simulink model "Distribution"  (R2018b)
settings: Solver=ode45  StartTime=0.0  StopTime=100  RelTol=1e-3
libraries: simeventslib x20
(part 2 of 2)

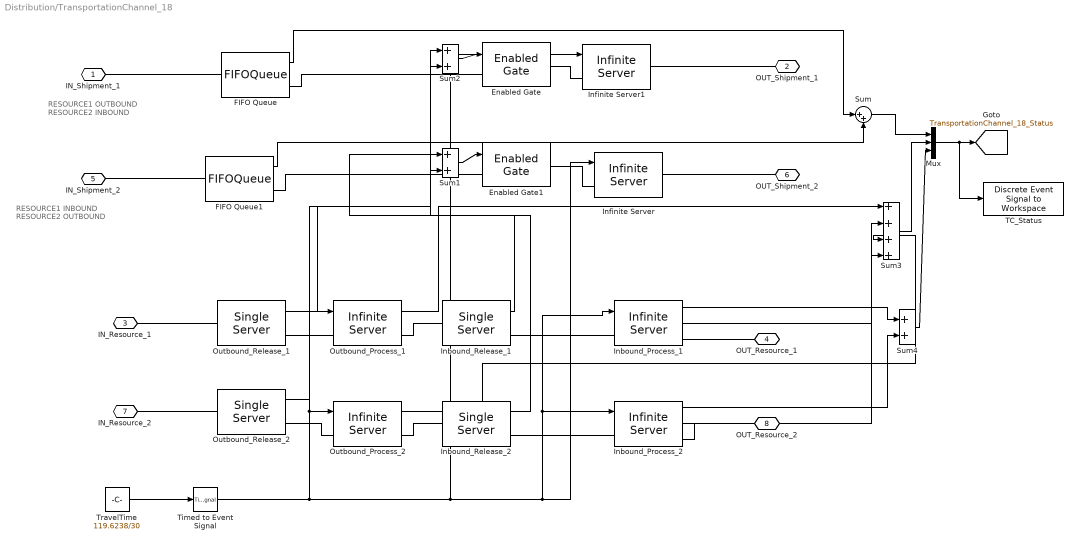
== system Distribution/TransportationChannel_18 ==
  note: RESOURCE1 OUTBOUND
      | RESOURCE2 INBOUND
  note: RESOURCE1 INBOUND
      | RESOURCE2 OUTBOUND
  Enabled Gate : EnabledGate
  Enabled Gate1 : EnabledGate
  FIFO Queue : FIFOQueue  Capacity=inf  StatNumberInBlock=on
      settings: OutputPortMap=o1
  FIFO Queue1 : FIFOQueue  Capacity=inf  StatNumberInBlock=on
      settings: OutputPortMap=o1
  Inbound_Process_1 : InfiniteServer  ServiceTimeFrom=Signal port t  ServiceTime=(76.7)/30  StatNumberDeparted=on  StatNumberInBlock=on
      settings: OutputPortMap=o0,o1
  Inbound_Process_2 : InfiniteServer  ServiceTimeFrom=Signal port t  ServiceTime=(76.7)/30  StatNumberDeparted=on  StatNumberInBlock=on
      settings: OutputPortMap=o0,o1
  Inbound_Release_1 : SingleServer  ServiceTime=0  StatNumberInBlock=on
      settings: OutputPortMap=o1
  Inbound_Release_2 : SingleServer  ServiceTime=0  StatNumberInBlock=on
      settings: OutputPortMap=o1
  Infinite Server : InfiniteServer  ServiceTimeFrom=Signal port t  ServiceTime=(76.7)/30
  Infinite Server1 : InfiniteServer  ServiceTimeFrom=Signal port t  ServiceTime=(76.7)/30
  Mux : Mux  Inputs=3
  Outbound_Process_1 : InfiniteServer  ServiceTimeFrom=Signal port t  ServiceTime=(76.7)/30  StatNumberInBlock=on
      settings: OutputPortMap=o1
  Outbound_Process_2 : InfiniteServer  ServiceTimeFrom=Signal port t  ServiceTime=(76.7)/30  StatNumberInBlock=on
      settings: OutputPortMap=o1
  Outbound_Release_1 : SingleServer  ServiceTime=0  StatNumberInBlock=on
      settings: OutputPortMap=o1
  Outbound_Release_2 : SingleServer  ServiceTime=0  StatNumberInBlock=on
      settings: OutputPortMap=o1
  Sum{,1..2,4} (4 alike) : Sum  Inputs=|++
  Sum3 : Sum  Inputs=|++++
  TC_Status : simeventslib/SimEvents Sinks/Discrete Event Signal to Workspace  VariableName=TransportationChannel_18_Status  SaveFormat=Structure With Time  isMonitorOnly=off  isRecordIC=off
      settings: SourceProductName=SimEvents  SourceProductBaseCode=SE
  Timed to Event Signal : TimedToEventSignal
  TravelTime : Constant  Value=119.6238/30
  IN_Shipment_1 : PMIOPort  Side=Left
  OUT_Shipment_1 : PMIOPort  Port=2  Side=Right
  IN_Resource_1 : PMIOPort  Port=3  Side=Left
  OUT_Resource_1 : PMIOPort  Port=4  Side=Right
  IN_Shipment_2 : PMIOPort  Port=5  Side=Left
  OUT_Shipment_2 : PMIOPort  Port=6  Side=Right
  IN_Resource_2 : PMIOPort  Port=7  Side=Left
  OUT_Resource_2 : PMIOPort  Port=8  Side=Right
  tag scope: TransportationChannel_18_Status=global
  wires:
  Sum4/1 -> Mux/3
  Inbound_Process_2/1 -> Sum4/2
  Inbound_Process_1/1 -> Sum4/1
  Inbound_Process_2/2 -> Sum3/4
  Outbound_Process_2/1 -> Sum3/3
  Inbound_Process_1/2 -> Sum3/2
  Outbound_Process_1/1 -> Sum3/1
  Sum3/1 -> Mux/2
  Sum/1 -> Mux/1
  Mux/1 -> TC_Status/1, [TransportationChannel_18_Status]
  Inbound_Release_2/1 -> Sum2/2
  Outbound_Release_1/1 -> Sum2/1
  Sum2/1 -> Enabled Gate/1
  Inbound_Release_1/1 -> Sum1/1
  Outbound_Release_2/1 -> Sum1/2
  Sum1/1 -> Enabled Gate1/1
  Timed to Event Signal/1 -> Outbound_Process_2/1, Outbound_Process_1/1, Infinite Server1/1, Inbound_Process_2/1, Inbound_Process_1/1, Infinite Server/1
  TravelTime/1 -> Timed to Event Signal/1
  FIFO Queue/1 -> Sum/1
  FIFO Queue1/1 -> Sum/2
  connections:
  Inbound_Process_1/RConn1 -- OUT_Resource_1/RConn1
  Outbound_Process_1/RConn1 -- Inbound_Release_1/LConn1
  Inbound_Release_1/RConn1 -- Inbound_Process_1/LConn1
  Outbound_Release_1/RConn1 -- Outbound_Process_1/LConn1
  Inbound_Process_2/RConn1 -- OUT_Resource_2/RConn1
  Inbound_Release_2/RConn1 -- Inbound_Process_2/LConn1
  Outbound_Process_2/RConn1 -- Inbound_Release_2/LConn1
  Outbound_Release_2/RConn1 -- Outbound_Process_2/LConn1
  IN_Resource_2/RConn1 -- Outbound_Release_2/LConn1
  Infinite Server1/RConn1 -- OUT_Shipment_1/RConn1
  Enabled Gate/RConn1 -- Infinite Server1/LConn1
  Infinite Server/LConn1 -- Enabled Gate1/RConn1
  OUT_Shipment_2/RConn1 -- Infinite Server/RConn1
  IN_Resource_1/RConn1 -- Outbound_Release_1/LConn1
  IN_Shipment_2/RConn1 -- FIFO Queue1/LConn1
  IN_Shipment_1/RConn1 -- FIFO Queue/LConn1
  Enabled Gate1/LConn1 -- FIFO Queue1/RConn1
  FIFO Queue/RConn1 -- Enabled Gate/LConn1

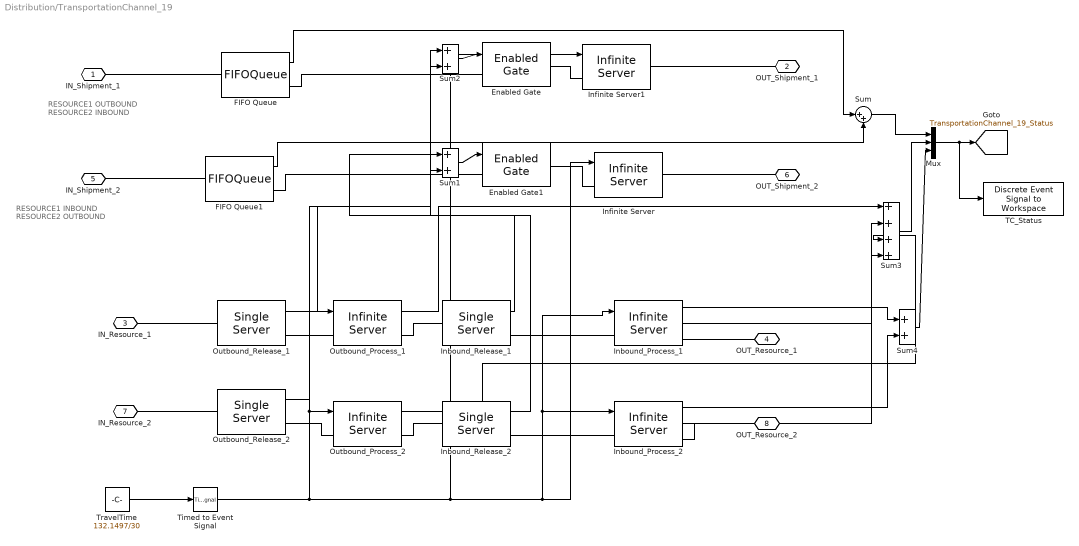
== system Distribution/TransportationChannel_19 ==
  note: RESOURCE1 OUTBOUND
      | RESOURCE2 INBOUND
  note: RESOURCE1 INBOUND
      | RESOURCE2 OUTBOUND
  Enabled Gate : EnabledGate
  Enabled Gate1 : EnabledGate
  FIFO Queue : FIFOQueue  Capacity=inf  StatNumberInBlock=on
      settings: OutputPortMap=o1
  FIFO Queue1 : FIFOQueue  Capacity=inf  StatNumberInBlock=on
      settings: OutputPortMap=o1
  Inbound_Process_1 : InfiniteServer  ServiceTimeFrom=Signal port t  ServiceTime=(76.7)/30  StatNumberDeparted=on  StatNumberInBlock=on
      settings: OutputPortMap=o0,o1
  Inbound_Process_2 : InfiniteServer  ServiceTimeFrom=Signal port t  ServiceTime=(76.7)/30  StatNumberDeparted=on  StatNumberInBlock=on
      settings: OutputPortMap=o0,o1
  Inbound_Release_1 : SingleServer  ServiceTime=0  StatNumberInBlock=on
      settings: OutputPortMap=o1
  Inbound_Release_2 : SingleServer  ServiceTime=0  StatNumberInBlock=on
      settings: OutputPortMap=o1
  Infinite Server : InfiniteServer  ServiceTimeFrom=Signal port t  ServiceTime=(76.7)/30
  Infinite Server1 : InfiniteServer  ServiceTimeFrom=Signal port t  ServiceTime=(76.7)/30
  Mux : Mux  Inputs=3
  Outbound_Process_1 : InfiniteServer  ServiceTimeFrom=Signal port t  ServiceTime=(76.7)/30  StatNumberInBlock=on
      settings: OutputPortMap=o1
  Outbound_Process_2 : InfiniteServer  ServiceTimeFrom=Signal port t  ServiceTime=(76.7)/30  StatNumberInBlock=on
      settings: OutputPortMap=o1
  Outbound_Release_1 : SingleServer  ServiceTime=0  StatNumberInBlock=on
      settings: OutputPortMap=o1
  Outbound_Release_2 : SingleServer  ServiceTime=0  StatNumberInBlock=on
      settings: OutputPortMap=o1
  Sum{,1..2,4} (4 alike) : Sum  Inputs=|++
  Sum3 : Sum  Inputs=|++++
  TC_Status : simeventslib/SimEvents Sinks/Discrete Event Signal to Workspace  VariableName=TransportationChannel_19_Status  SaveFormat=Structure With Time  isMonitorOnly=off  isRecordIC=off
      settings: SourceProductName=SimEvents  SourceProductBaseCode=SE
  Timed to Event Signal : TimedToEventSignal
  TravelTime : Constant  Value=132.1497/30
  IN_Shipment_1 : PMIOPort  Side=Left
  OUT_Shipment_1 : PMIOPort  Port=2  Side=Right
  IN_Resource_1 : PMIOPort  Port=3  Side=Left
  OUT_Resource_1 : PMIOPort  Port=4  Side=Right
  IN_Shipment_2 : PMIOPort  Port=5  Side=Left
  OUT_Shipment_2 : PMIOPort  Port=6  Side=Right
  IN_Resource_2 : PMIOPort  Port=7  Side=Left
  OUT_Resource_2 : PMIOPort  Port=8  Side=Right
  tag scope: TransportationChannel_19_Status=global
  wires:
  Sum4/1 -> Mux/3
  Inbound_Process_2/1 -> Sum4/2
  Inbound_Process_1/1 -> Sum4/1
  Inbound_Process_2/2 -> Sum3/4
  Outbound_Process_2/1 -> Sum3/3
  Inbound_Process_1/2 -> Sum3/2
  Outbound_Process_1/1 -> Sum3/1
  Sum3/1 -> Mux/2
  Sum/1 -> Mux/1
  Mux/1 -> TC_Status/1, [TransportationChannel_19_Status]
  Inbound_Release_2/1 -> Sum2/2
  Outbound_Release_1/1 -> Sum2/1
  Sum2/1 -> Enabled Gate/1
  Inbound_Release_1/1 -> Sum1/1
  Outbound_Release_2/1 -> Sum1/2
  Sum1/1 -> Enabled Gate1/1
  Timed to Event Signal/1 -> Outbound_Process_2/1, Outbound_Process_1/1, Infinite Server1/1, Inbound_Process_2/1, Inbound_Process_1/1, Infinite Server/1
  TravelTime/1 -> Timed to Event Signal/1
  FIFO Queue/1 -> Sum/1
  FIFO Queue1/1 -> Sum/2
  connections:
  Inbound_Process_1/RConn1 -- OUT_Resource_1/RConn1
  Outbound_Process_1/RConn1 -- Inbound_Release_1/LConn1
  Inbound_Release_1/RConn1 -- Inbound_Process_1/LConn1
  Outbound_Release_1/RConn1 -- Outbound_Process_1/LConn1
  Inbound_Process_2/RConn1 -- OUT_Resource_2/RConn1
  Inbound_Release_2/RConn1 -- Inbound_Process_2/LConn1
  Outbound_Process_2/RConn1 -- Inbound_Release_2/LConn1
  Outbound_Release_2/RConn1 -- Outbound_Process_2/LConn1
  IN_Resource_2/RConn1 -- Outbound_Release_2/LConn1
  Infinite Server1/RConn1 -- OUT_Shipment_1/RConn1
  Enabled Gate/RConn1 -- Infinite Server1/LConn1
  Infinite Server/LConn1 -- Enabled Gate1/RConn1
  OUT_Shipment_2/RConn1 -- Infinite Server/RConn1
  IN_Resource_1/RConn1 -- Outbound_Release_1/LConn1
  IN_Shipment_2/RConn1 -- FIFO Queue1/LConn1
  IN_Shipment_1/RConn1 -- FIFO Queue/LConn1
  Enabled Gate1/LConn1 -- FIFO Queue1/RConn1
  FIFO Queue/RConn1 -- Enabled Gate/LConn1

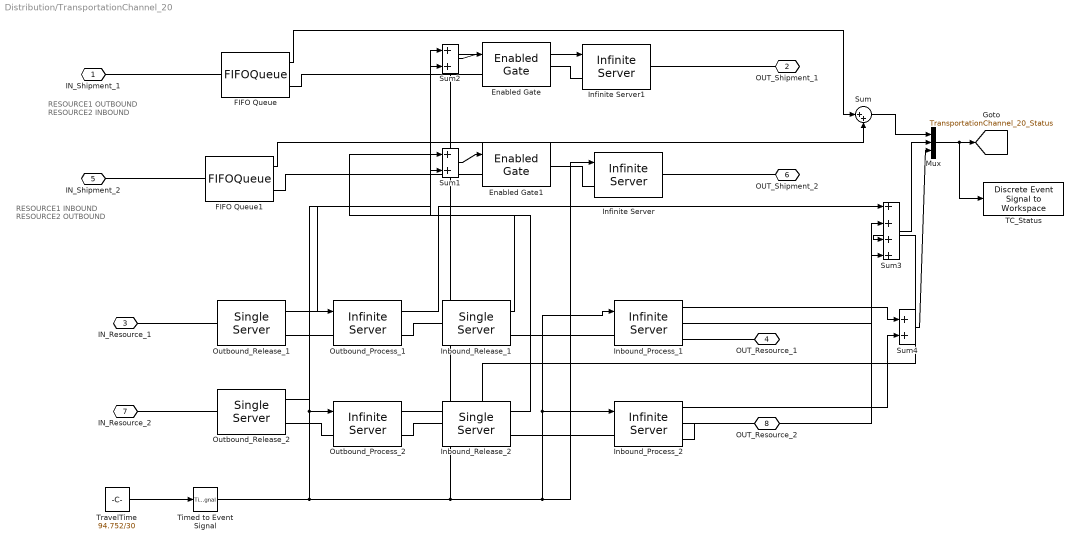
== system Distribution/TransportationChannel_20 ==
  note: RESOURCE1 OUTBOUND
      | RESOURCE2 INBOUND
  note: RESOURCE1 INBOUND
      | RESOURCE2 OUTBOUND
  Enabled Gate : EnabledGate
  Enabled Gate1 : EnabledGate
  FIFO Queue : FIFOQueue  Capacity=inf  StatNumberInBlock=on
      settings: OutputPortMap=o1
  FIFO Queue1 : FIFOQueue  Capacity=inf  StatNumberInBlock=on
      settings: OutputPortMap=o1
  Inbound_Process_1 : InfiniteServer  ServiceTimeFrom=Signal port t  ServiceTime=(76.7)/30  StatNumberDeparted=on  StatNumberInBlock=on
      settings: OutputPortMap=o0,o1
  Inbound_Process_2 : InfiniteServer  ServiceTimeFrom=Signal port t  ServiceTime=(76.7)/30  StatNumberDeparted=on  StatNumberInBlock=on
      settings: OutputPortMap=o0,o1
  Inbound_Release_1 : SingleServer  ServiceTime=0  StatNumberInBlock=on
      settings: OutputPortMap=o1
  Inbound_Release_2 : SingleServer  ServiceTime=0  StatNumberInBlock=on
      settings: OutputPortMap=o1
  Infinite Server : InfiniteServer  ServiceTimeFrom=Signal port t  ServiceTime=(76.7)/30
  Infinite Server1 : InfiniteServer  ServiceTimeFrom=Signal port t  ServiceTime=(76.7)/30
  Mux : Mux  Inputs=3
  Outbound_Process_1 : InfiniteServer  ServiceTimeFrom=Signal port t  ServiceTime=(76.7)/30  StatNumberInBlock=on
      settings: OutputPortMap=o1
  Outbound_Process_2 : InfiniteServer  ServiceTimeFrom=Signal port t  ServiceTime=(76.7)/30  StatNumberInBlock=on
      settings: OutputPortMap=o1
  Outbound_Release_1 : SingleServer  ServiceTime=0  StatNumberInBlock=on
      settings: OutputPortMap=o1
  Outbound_Release_2 : SingleServer  ServiceTime=0  StatNumberInBlock=on
      settings: OutputPortMap=o1
  Sum{,1..2,4} (4 alike) : Sum  Inputs=|++
  Sum3 : Sum  Inputs=|++++
  TC_Status : simeventslib/SimEvents Sinks/Discrete Event Signal to Workspace  VariableName=TransportationChannel_20_Status  SaveFormat=Structure With Time  isMonitorOnly=off  isRecordIC=off
      settings: SourceProductName=SimEvents  SourceProductBaseCode=SE
  Timed to Event Signal : TimedToEventSignal
  TravelTime : Constant  Value=94.752/30
  IN_Shipment_1 : PMIOPort  Side=Left
  OUT_Shipment_1 : PMIOPort  Port=2  Side=Right
  IN_Resource_1 : PMIOPort  Port=3  Side=Left
  OUT_Resource_1 : PMIOPort  Port=4  Side=Right
  IN_Shipment_2 : PMIOPort  Port=5  Side=Left
  OUT_Shipment_2 : PMIOPort  Port=6  Side=Right
  IN_Resource_2 : PMIOPort  Port=7  Side=Left
  OUT_Resource_2 : PMIOPort  Port=8  Side=Right
  tag scope: TransportationChannel_20_Status=global
  wires:
  Sum4/1 -> Mux/3
  Inbound_Process_2/1 -> Sum4/2
  Inbound_Process_1/1 -> Sum4/1
  Inbound_Process_2/2 -> Sum3/4
  Outbound_Process_2/1 -> Sum3/3
  Inbound_Process_1/2 -> Sum3/2
  Outbound_Process_1/1 -> Sum3/1
  Sum3/1 -> Mux/2
  Sum/1 -> Mux/1
  Mux/1 -> TC_Status/1, [TransportationChannel_20_Status]
  Inbound_Release_2/1 -> Sum2/2
  Outbound_Release_1/1 -> Sum2/1
  Sum2/1 -> Enabled Gate/1
  Inbound_Release_1/1 -> Sum1/1
  Outbound_Release_2/1 -> Sum1/2
  Sum1/1 -> Enabled Gate1/1
  Timed to Event Signal/1 -> Outbound_Process_2/1, Outbound_Process_1/1, Infinite Server1/1, Inbound_Process_2/1, Inbound_Process_1/1, Infinite Server/1
  TravelTime/1 -> Timed to Event Signal/1
  FIFO Queue/1 -> Sum/1
  FIFO Queue1/1 -> Sum/2
  connections:
  Inbound_Process_1/RConn1 -- OUT_Resource_1/RConn1
  Outbound_Process_1/RConn1 -- Inbound_Release_1/LConn1
  Inbound_Release_1/RConn1 -- Inbound_Process_1/LConn1
  Outbound_Release_1/RConn1 -- Outbound_Process_1/LConn1
  Inbound_Process_2/RConn1 -- OUT_Resource_2/RConn1
  Inbound_Release_2/RConn1 -- Inbound_Process_2/LConn1
  Outbound_Process_2/RConn1 -- Inbound_Release_2/LConn1
  Outbound_Release_2/RConn1 -- Outbound_Process_2/LConn1
  IN_Resource_2/RConn1 -- Outbound_Release_2/LConn1
  Infinite Server1/RConn1 -- OUT_Shipment_1/RConn1
  Enabled Gate/RConn1 -- Infinite Server1/LConn1
  Infinite Server/LConn1 -- Enabled Gate1/RConn1
  OUT_Shipment_2/RConn1 -- Infinite Server/RConn1
  IN_Resource_1/RConn1 -- Outbound_Release_1/LConn1
  IN_Shipment_2/RConn1 -- FIFO Queue1/LConn1
  IN_Shipment_1/RConn1 -- FIFO Queue/LConn1
  Enabled Gate1/LConn1 -- FIFO Queue1/RConn1
  FIFO Queue/RConn1 -- Enabled Gate/LConn1

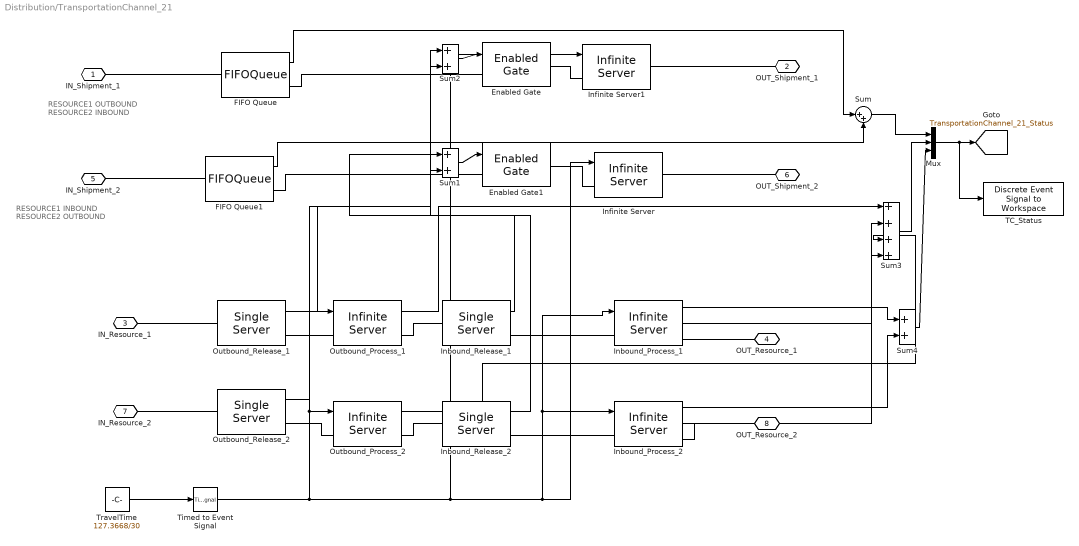
== system Distribution/TransportationChannel_21 ==
  note: RESOURCE1 OUTBOUND
      | RESOURCE2 INBOUND
  note: RESOURCE1 INBOUND
      | RESOURCE2 OUTBOUND
  Enabled Gate : EnabledGate
  Enabled Gate1 : EnabledGate
  FIFO Queue : FIFOQueue  Capacity=inf  StatNumberInBlock=on
      settings: OutputPortMap=o1
  FIFO Queue1 : FIFOQueue  Capacity=inf  StatNumberInBlock=on
      settings: OutputPortMap=o1
  Inbound_Process_1 : InfiniteServer  ServiceTimeFrom=Signal port t  ServiceTime=(76.7)/30  StatNumberDeparted=on  StatNumberInBlock=on
      settings: OutputPortMap=o0,o1
  Inbound_Process_2 : InfiniteServer  ServiceTimeFrom=Signal port t  ServiceTime=(76.7)/30  StatNumberDeparted=on  StatNumberInBlock=on
      settings: OutputPortMap=o0,o1
  Inbound_Release_1 : SingleServer  ServiceTime=0  StatNumberInBlock=on
      settings: OutputPortMap=o1
  Inbound_Release_2 : SingleServer  ServiceTime=0  StatNumberInBlock=on
      settings: OutputPortMap=o1
  Infinite Server : InfiniteServer  ServiceTimeFrom=Signal port t  ServiceTime=(76.7)/30
  Infinite Server1 : InfiniteServer  ServiceTimeFrom=Signal port t  ServiceTime=(76.7)/30
  Mux : Mux  Inputs=3
  Outbound_Process_1 : InfiniteServer  ServiceTimeFrom=Signal port t  ServiceTime=(76.7)/30  StatNumberInBlock=on
      settings: OutputPortMap=o1
  Outbound_Process_2 : InfiniteServer  ServiceTimeFrom=Signal port t  ServiceTime=(76.7)/30  StatNumberInBlock=on
      settings: OutputPortMap=o1
  Outbound_Release_1 : SingleServer  ServiceTime=0  StatNumberInBlock=on
      settings: OutputPortMap=o1
  Outbound_Release_2 : SingleServer  ServiceTime=0  StatNumberInBlock=on
      settings: OutputPortMap=o1
  Sum{,1..2,4} (4 alike) : Sum  Inputs=|++
  Sum3 : Sum  Inputs=|++++
  TC_Status : simeventslib/SimEvents Sinks/Discrete Event Signal to Workspace  VariableName=TransportationChannel_21_Status  SaveFormat=Structure With Time  isMonitorOnly=off  isRecordIC=off
      settings: SourceProductName=SimEvents  SourceProductBaseCode=SE
  Timed to Event Signal : TimedToEventSignal
  TravelTime : Constant  Value=127.3668/30
  IN_Shipment_1 : PMIOPort  Side=Left
  OUT_Shipment_1 : PMIOPort  Port=2  Side=Right
  IN_Resource_1 : PMIOPort  Port=3  Side=Left
  OUT_Resource_1 : PMIOPort  Port=4  Side=Right
  IN_Shipment_2 : PMIOPort  Port=5  Side=Left
  OUT_Shipment_2 : PMIOPort  Port=6  Side=Right
  IN_Resource_2 : PMIOPort  Port=7  Side=Left
  OUT_Resource_2 : PMIOPort  Port=8  Side=Right
  tag scope: TransportationChannel_21_Status=global
  wires:
  Sum4/1 -> Mux/3
  Inbound_Process_2/1 -> Sum4/2
  Inbound_Process_1/1 -> Sum4/1
  Inbound_Process_2/2 -> Sum3/4
  Outbound_Process_2/1 -> Sum3/3
  Inbound_Process_1/2 -> Sum3/2
  Outbound_Process_1/1 -> Sum3/1
  Sum3/1 -> Mux/2
  Sum/1 -> Mux/1
  Mux/1 -> TC_Status/1, [TransportationChannel_21_Status]
  Inbound_Release_2/1 -> Sum2/2
  Outbound_Release_1/1 -> Sum2/1
  Sum2/1 -> Enabled Gate/1
  Inbound_Release_1/1 -> Sum1/1
  Outbound_Release_2/1 -> Sum1/2
  Sum1/1 -> Enabled Gate1/1
  Timed to Event Signal/1 -> Outbound_Process_2/1, Outbound_Process_1/1, Infinite Server1/1, Inbound_Process_2/1, Inbound_Process_1/1, Infinite Server/1
  TravelTime/1 -> Timed to Event Signal/1
  FIFO Queue/1 -> Sum/1
  FIFO Queue1/1 -> Sum/2
  connections:
  Inbound_Process_1/RConn1 -- OUT_Resource_1/RConn1
  Outbound_Process_1/RConn1 -- Inbound_Release_1/LConn1
  Inbound_Release_1/RConn1 -- Inbound_Process_1/LConn1
  Outbound_Release_1/RConn1 -- Outbound_Process_1/LConn1
  Inbound_Process_2/RConn1 -- OUT_Resource_2/RConn1
  Inbound_Release_2/RConn1 -- Inbound_Process_2/LConn1
  Outbound_Process_2/RConn1 -- Inbound_Release_2/LConn1
  Outbound_Release_2/RConn1 -- Outbound_Process_2/LConn1
  IN_Resource_2/RConn1 -- Outbound_Release_2/LConn1
  Infinite Server1/RConn1 -- OUT_Shipment_1/RConn1
  Enabled Gate/RConn1 -- Infinite Server1/LConn1
  Infinite Server/LConn1 -- Enabled Gate1/RConn1
  OUT_Shipment_2/RConn1 -- Infinite Server/RConn1
  IN_Resource_1/RConn1 -- Outbound_Release_1/LConn1
  IN_Shipment_2/RConn1 -- FIFO Queue1/LConn1
  IN_Shipment_1/RConn1 -- FIFO Queue/LConn1
  Enabled Gate1/LConn1 -- FIFO Queue1/RConn1
  FIFO Queue/RConn1 -- Enabled Gate/LConn1

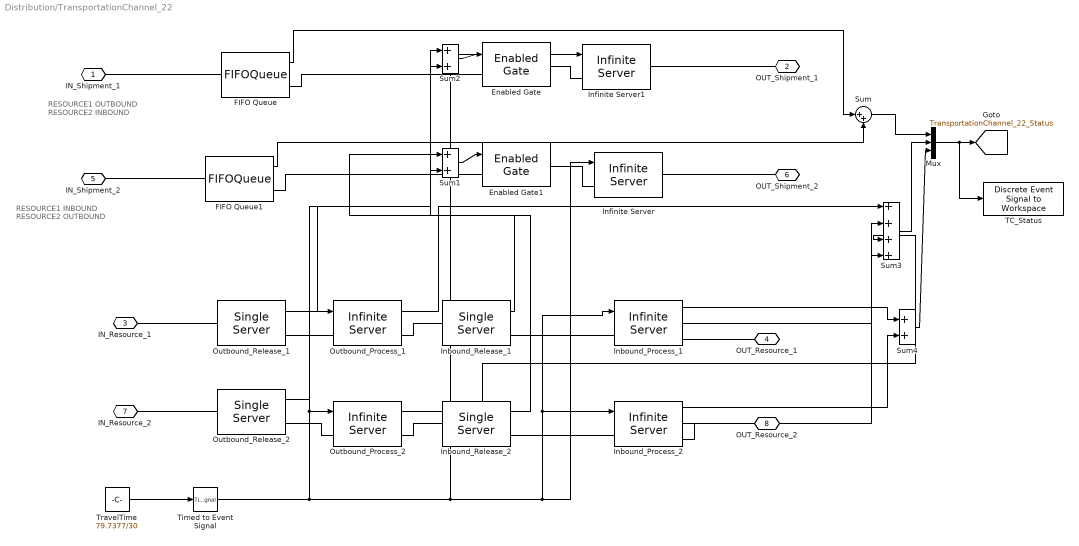
== system Distribution/TransportationChannel_22 ==
  note: RESOURCE1 OUTBOUND
      | RESOURCE2 INBOUND
  note: RESOURCE1 INBOUND
      | RESOURCE2 OUTBOUND
  Enabled Gate : EnabledGate
  Enabled Gate1 : EnabledGate
  FIFO Queue : FIFOQueue  Capacity=inf  StatNumberInBlock=on
      settings: OutputPortMap=o1
  FIFO Queue1 : FIFOQueue  Capacity=inf  StatNumberInBlock=on
      settings: OutputPortMap=o1
  Inbound_Process_1 : InfiniteServer  ServiceTimeFrom=Signal port t  ServiceTime=(76.7)/30  StatNumberDeparted=on  StatNumberInBlock=on
      settings: OutputPortMap=o0,o1
  Inbound_Process_2 : InfiniteServer  ServiceTimeFrom=Signal port t  ServiceTime=(76.7)/30  StatNumberDeparted=on  StatNumberInBlock=on
      settings: OutputPortMap=o0,o1
  Inbound_Release_1 : SingleServer  ServiceTime=0  StatNumberInBlock=on
      settings: OutputPortMap=o1
  Inbound_Release_2 : SingleServer  ServiceTime=0  StatNumberInBlock=on
      settings: OutputPortMap=o1
  Infinite Server : InfiniteServer  ServiceTimeFrom=Signal port t  ServiceTime=(76.7)/30
  Infinite Server1 : InfiniteServer  ServiceTimeFrom=Signal port t  ServiceTime=(76.7)/30
  Mux : Mux  Inputs=3
  Outbound_Process_1 : InfiniteServer  ServiceTimeFrom=Signal port t  ServiceTime=(76.7)/30  StatNumberInBlock=on
      settings: OutputPortMap=o1
  Outbound_Process_2 : InfiniteServer  ServiceTimeFrom=Signal port t  ServiceTime=(76.7)/30  StatNumberInBlock=on
      settings: OutputPortMap=o1
  Outbound_Release_1 : SingleServer  ServiceTime=0  StatNumberInBlock=on
      settings: OutputPortMap=o1
  Outbound_Release_2 : SingleServer  ServiceTime=0  StatNumberInBlock=on
      settings: OutputPortMap=o1
  Sum{,1..2,4} (4 alike) : Sum  Inputs=|++
  Sum3 : Sum  Inputs=|++++
  TC_Status : simeventslib/SimEvents Sinks/Discrete Event Signal to Workspace  VariableName=TransportationChannel_22_Status  SaveFormat=Structure With Time  isMonitorOnly=off  isRecordIC=off
      settings: SourceProductName=SimEvents  SourceProductBaseCode=SE
  Timed to Event Signal : TimedToEventSignal
  TravelTime : Constant  Value=79.7377/30
  IN_Shipment_1 : PMIOPort  Side=Left
  OUT_Shipment_1 : PMIOPort  Port=2  Side=Right
  IN_Resource_1 : PMIOPort  Port=3  Side=Left
  OUT_Resource_1 : PMIOPort  Port=4  Side=Right
  IN_Shipment_2 : PMIOPort  Port=5  Side=Left
  OUT_Shipment_2 : PMIOPort  Port=6  Side=Right
  IN_Resource_2 : PMIOPort  Port=7  Side=Left
  OUT_Resource_2 : PMIOPort  Port=8  Side=Right
  tag scope: TransportationChannel_22_Status=global
  wires:
  Sum4/1 -> Mux/3
  Inbound_Process_2/1 -> Sum4/2
  Inbound_Process_1/1 -> Sum4/1
  Inbound_Process_2/2 -> Sum3/4
  Outbound_Process_2/1 -> Sum3/3
  Inbound_Process_1/2 -> Sum3/2
  Outbound_Process_1/1 -> Sum3/1
  Sum3/1 -> Mux/2
  Sum/1 -> Mux/1
  Mux/1 -> TC_Status/1, [TransportationChannel_22_Status]
  Inbound_Release_2/1 -> Sum2/2
  Outbound_Release_1/1 -> Sum2/1
  Sum2/1 -> Enabled Gate/1
  Inbound_Release_1/1 -> Sum1/1
  Outbound_Release_2/1 -> Sum1/2
  Sum1/1 -> Enabled Gate1/1
  Timed to Event Signal/1 -> Outbound_Process_2/1, Outbound_Process_1/1, Infinite Server1/1, Inbound_Process_2/1, Inbound_Process_1/1, Infinite Server/1
  TravelTime/1 -> Timed to Event Signal/1
  FIFO Queue/1 -> Sum/1
  FIFO Queue1/1 -> Sum/2
  connections:
  Inbound_Process_1/RConn1 -- OUT_Resource_1/RConn1
  Outbound_Process_1/RConn1 -- Inbound_Release_1/LConn1
  Inbound_Release_1/RConn1 -- Inbound_Process_1/LConn1
  Outbound_Release_1/RConn1 -- Outbound_Process_1/LConn1
  Inbound_Process_2/RConn1 -- OUT_Resource_2/RConn1
  Inbound_Release_2/RConn1 -- Inbound_Process_2/LConn1
  Outbound_Process_2/RConn1 -- Inbound_Release_2/LConn1
  Outbound_Release_2/RConn1 -- Outbound_Process_2/LConn1
  IN_Resource_2/RConn1 -- Outbound_Release_2/LConn1
  Infinite Server1/RConn1 -- OUT_Shipment_1/RConn1
  Enabled Gate/RConn1 -- Infinite Server1/LConn1
  Infinite Server/LConn1 -- Enabled Gate1/RConn1
  OUT_Shipment_2/RConn1 -- Infinite Server/RConn1
  IN_Resource_1/RConn1 -- Outbound_Release_1/LConn1
  IN_Shipment_2/RConn1 -- FIFO Queue1/LConn1
  IN_Shipment_1/RConn1 -- FIFO Queue/LConn1
  Enabled Gate1/LConn1 -- FIFO Queue1/RConn1
  FIFO Queue/RConn1 -- Enabled Gate/LConn1

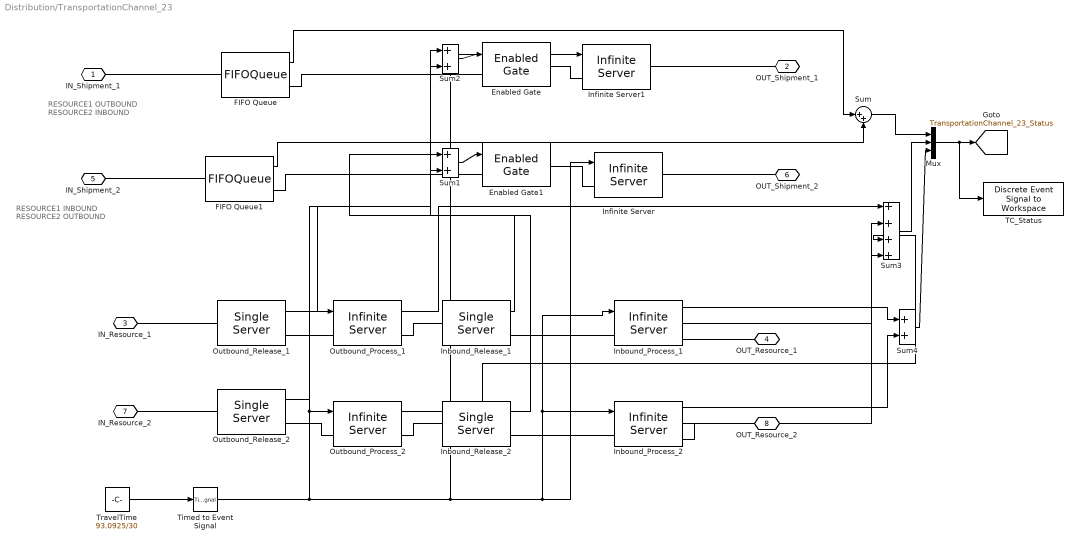
== system Distribution/TransportationChannel_23 ==
  note: RESOURCE1 OUTBOUND
      | RESOURCE2 INBOUND
  note: RESOURCE1 INBOUND
      | RESOURCE2 OUTBOUND
  Enabled Gate : EnabledGate
  Enabled Gate1 : EnabledGate
  FIFO Queue : FIFOQueue  Capacity=inf  StatNumberInBlock=on
      settings: OutputPortMap=o1
  FIFO Queue1 : FIFOQueue  Capacity=inf  StatNumberInBlock=on
      settings: OutputPortMap=o1
  Inbound_Process_1 : InfiniteServer  ServiceTimeFrom=Signal port t  ServiceTime=(76.7)/30  StatNumberDeparted=on  StatNumberInBlock=on
      settings: OutputPortMap=o0,o1
  Inbound_Process_2 : InfiniteServer  ServiceTimeFrom=Signal port t  ServiceTime=(76.7)/30  StatNumberDeparted=on  StatNumberInBlock=on
      settings: OutputPortMap=o0,o1
  Inbound_Release_1 : SingleServer  ServiceTime=0  StatNumberInBlock=on
      settings: OutputPortMap=o1
  Inbound_Release_2 : SingleServer  ServiceTime=0  StatNumberInBlock=on
      settings: OutputPortMap=o1
  Infinite Server : InfiniteServer  ServiceTimeFrom=Signal port t  ServiceTime=(76.7)/30
  Infinite Server1 : InfiniteServer  ServiceTimeFrom=Signal port t  ServiceTime=(76.7)/30
  Mux : Mux  Inputs=3
  Outbound_Process_1 : InfiniteServer  ServiceTimeFrom=Signal port t  ServiceTime=(76.7)/30  StatNumberInBlock=on
      settings: OutputPortMap=o1
  Outbound_Process_2 : InfiniteServer  ServiceTimeFrom=Signal port t  ServiceTime=(76.7)/30  StatNumberInBlock=on
      settings: OutputPortMap=o1
  Outbound_Release_1 : SingleServer  ServiceTime=0  StatNumberInBlock=on
      settings: OutputPortMap=o1
  Outbound_Release_2 : SingleServer  ServiceTime=0  StatNumberInBlock=on
      settings: OutputPortMap=o1
  Sum{,1..2,4} (4 alike) : Sum  Inputs=|++
  Sum3 : Sum  Inputs=|++++
  TC_Status : simeventslib/SimEvents Sinks/Discrete Event Signal to Workspace  VariableName=TransportationChannel_23_Status  SaveFormat=Structure With Time  isMonitorOnly=off  isRecordIC=off
      settings: SourceProductName=SimEvents  SourceProductBaseCode=SE
  Timed to Event Signal : TimedToEventSignal
  TravelTime : Constant  Value=93.0925/30
  IN_Shipment_1 : PMIOPort  Side=Left
  OUT_Shipment_1 : PMIOPort  Port=2  Side=Right
  IN_Resource_1 : PMIOPort  Port=3  Side=Left
  OUT_Resource_1 : PMIOPort  Port=4  Side=Right
  IN_Shipment_2 : PMIOPort  Port=5  Side=Left
  OUT_Shipment_2 : PMIOPort  Port=6  Side=Right
  IN_Resource_2 : PMIOPort  Port=7  Side=Left
  OUT_Resource_2 : PMIOPort  Port=8  Side=Right
  tag scope: TransportationChannel_23_Status=global
  wires:
  Sum4/1 -> Mux/3
  Inbound_Process_2/1 -> Sum4/2
  Inbound_Process_1/1 -> Sum4/1
  Inbound_Process_2/2 -> Sum3/4
  Outbound_Process_2/1 -> Sum3/3
  Inbound_Process_1/2 -> Sum3/2
  Outbound_Process_1/1 -> Sum3/1
  Sum3/1 -> Mux/2
  Sum/1 -> Mux/1
  Mux/1 -> TC_Status/1, [TransportationChannel_23_Status]
  Inbound_Release_2/1 -> Sum2/2
  Outbound_Release_1/1 -> Sum2/1
  Sum2/1 -> Enabled Gate/1
  Inbound_Release_1/1 -> Sum1/1
  Outbound_Release_2/1 -> Sum1/2
  Sum1/1 -> Enabled Gate1/1
  Timed to Event Signal/1 -> Outbound_Process_2/1, Outbound_Process_1/1, Infinite Server1/1, Inbound_Process_2/1, Inbound_Process_1/1, Infinite Server/1
  TravelTime/1 -> Timed to Event Signal/1
  FIFO Queue/1 -> Sum/1
  FIFO Queue1/1 -> Sum/2
  connections:
  Inbound_Process_1/RConn1 -- OUT_Resource_1/RConn1
  Outbound_Process_1/RConn1 -- Inbound_Release_1/LConn1
  Inbound_Release_1/RConn1 -- Inbound_Process_1/LConn1
  Outbound_Release_1/RConn1 -- Outbound_Process_1/LConn1
  Inbound_Process_2/RConn1 -- OUT_Resource_2/RConn1
  Inbound_Release_2/RConn1 -- Inbound_Process_2/LConn1
  Outbound_Process_2/RConn1 -- Inbound_Release_2/LConn1
  Outbound_Release_2/RConn1 -- Outbound_Process_2/LConn1
  IN_Resource_2/RConn1 -- Outbound_Release_2/LConn1
  Infinite Server1/RConn1 -- OUT_Shipment_1/RConn1
  Enabled Gate/RConn1 -- Infinite Server1/LConn1
  Infinite Server/LConn1 -- Enabled Gate1/RConn1
  OUT_Shipment_2/RConn1 -- Infinite Server/RConn1
  IN_Resource_1/RConn1 -- Outbound_Release_1/LConn1
  IN_Shipment_2/RConn1 -- FIFO Queue1/LConn1
  IN_Shipment_1/RConn1 -- FIFO Queue/LConn1
  Enabled Gate1/LConn1 -- FIFO Queue1/RConn1
  FIFO Queue/RConn1 -- Enabled Gate/LConn1

== system Distribution/Customer1/AggregateCommodity ==
  Clock : Clock
  Source : TimeBasedEntityGenerator  Distribution=Exponential  InitialSeed=27167  Mean=Mean  GenerateEntityAtSimulationStart=off
  Timed to Event Signal : TimedToEventSignal
  setAttribute : SetAttribute  AttributeName=Route|Origin|Destination|Start  AttributeFrom=Dialog|Dialog|Dialog|Signal port  AttributeValue=[1 0 1]|1|1|1  AttributeTreatAsVector=0|1|1|1  EvaluatedAttributeValue={ [1 0 1];1;1;[]}
      settings: InputPortMap=u3
  OUT_Commodity : PMIOPort  Side=Right
  wires:
  Timed to Event Signal/1 -> setAttribute/1
  Clock/1 -> Timed to Event Signal/1
  connections:
  OUT_Commodity/RConn1 -- setAttribute/RConn1
  Source/RConn1 -- setAttribute/LConn1

== system Distribution/Customer10/AggregateCommodity ==
  Clock : Clock
  Source : TimeBasedEntityGenerator  Distribution=Exponential  InitialSeed=30384  Mean=Mean  GenerateEntityAtSimulationStart=off
  Timed to Event Signal : TimedToEventSignal
  setAttribute : SetAttribute  AttributeName=Route|Origin|Destination|Start  AttributeFrom=Dialog|Dialog|Dialog|Signal port  AttributeValue=[1 0 1]|1|1|1  AttributeTreatAsVector=0|1|1|1  EvaluatedAttributeValue={ [1 0 1];1;1;[]}
      settings: InputPortMap=u3
  OUT_Commodity : PMIOPort  Side=Right
  wires:
  Timed to Event Signal/1 -> setAttribute/1
  Clock/1 -> Timed to Event Signal/1
  connections:
  OUT_Commodity/RConn1 -- setAttribute/RConn1
  Source/RConn1 -- setAttribute/LConn1

== system Distribution/Customer2/AggregateCommodity ==
  Clock : Clock
  Source : TimeBasedEntityGenerator  Distribution=Exponential  InitialSeed=33601  Mean=Mean  GenerateEntityAtSimulationStart=off
  Timed to Event Signal : TimedToEventSignal
  setAttribute : SetAttribute  AttributeName=Route|Origin|Destination|Start  AttributeFrom=Dialog|Dialog|Dialog|Signal port  AttributeValue=[1 0 1]|1|1|1  AttributeTreatAsVector=0|1|1|1  EvaluatedAttributeValue={ [1 0 1];1;1;[]}
      settings: InputPortMap=u3
  OUT_Commodity : PMIOPort  Side=Right
  wires:
  Timed to Event Signal/1 -> setAttribute/1
  Clock/1 -> Timed to Event Signal/1
  connections:
  OUT_Commodity/RConn1 -- setAttribute/RConn1
  Source/RConn1 -- setAttribute/LConn1

== system Distribution/Customer3/AggregateCommodity ==
  Clock : Clock
  Source : TimeBasedEntityGenerator  Distribution=Exponential  InitialSeed=36818  Mean=Mean  GenerateEntityAtSimulationStart=off
  Timed to Event Signal : TimedToEventSignal
  setAttribute : SetAttribute  AttributeName=Route|Origin|Destination|Start  AttributeFrom=Dialog|Dialog|Dialog|Signal port  AttributeValue=[1 0 1]|1|1|1  AttributeTreatAsVector=0|1|1|1  EvaluatedAttributeValue={ [1 0 1];1;1;[]}
      settings: InputPortMap=u3
  OUT_Commodity : PMIOPort  Side=Right
  wires:
  Timed to Event Signal/1 -> setAttribute/1
  Clock/1 -> Timed to Event Signal/1
  connections:
  OUT_Commodity/RConn1 -- setAttribute/RConn1
  Source/RConn1 -- setAttribute/LConn1

== system Distribution/Customer4/AggregateCommodity ==
  Clock : Clock
  Source : TimeBasedEntityGenerator  Distribution=Exponential  InitialSeed=40035  Mean=Mean  GenerateEntityAtSimulationStart=off
  Timed to Event Signal : TimedToEventSignal
  setAttribute : SetAttribute  AttributeName=Route|Origin|Destination|Start  AttributeFrom=Dialog|Dialog|Dialog|Signal port  AttributeValue=[1 0 1]|1|1|1  AttributeTreatAsVector=0|1|1|1  EvaluatedAttributeValue={ [1 0 1];1;1;[]}
      settings: InputPortMap=u3
  OUT_Commodity : PMIOPort  Side=Right
  wires:
  Timed to Event Signal/1 -> setAttribute/1
  Clock/1 -> Timed to Event Signal/1
  connections:
  OUT_Commodity/RConn1 -- setAttribute/RConn1
  Source/RConn1 -- setAttribute/LConn1

== system Distribution/Customer5/AggregateCommodity ==
  Clock : Clock
  Source : TimeBasedEntityGenerator  Distribution=Exponential  InitialSeed=43252  Mean=Mean  GenerateEntityAtSimulationStart=off
  Timed to Event Signal : TimedToEventSignal
  setAttribute : SetAttribute  AttributeName=Route|Origin|Destination|Start  AttributeFrom=Dialog|Dialog|Dialog|Signal port  AttributeValue=[1 0 1]|1|1|1  AttributeTreatAsVector=0|1|1|1  EvaluatedAttributeValue={ [1 0 1];1;1;[]}
      settings: InputPortMap=u3
  OUT_Commodity : PMIOPort  Side=Right
  wires:
  Timed to Event Signal/1 -> setAttribute/1
  Clock/1 -> Timed to Event Signal/1
  connections:
  OUT_Commodity/RConn1 -- setAttribute/RConn1
  Source/RConn1 -- setAttribute/LConn1

== system Distribution/Customer6/AggregateCommodity ==
  Clock : Clock
  Source : TimeBasedEntityGenerator  Distribution=Exponential  InitialSeed=46469  Mean=Mean  GenerateEntityAtSimulationStart=off
  Timed to Event Signal : TimedToEventSignal
  setAttribute : SetAttribute  AttributeName=Route|Origin|Destination|Start  AttributeFrom=Dialog|Dialog|Dialog|Signal port  AttributeValue=[1 0 1]|1|1|1  AttributeTreatAsVector=0|1|1|1  EvaluatedAttributeValue={ [1 0 1];1;1;[]}
      settings: InputPortMap=u3
  OUT_Commodity : PMIOPort  Side=Right
  wires:
  Timed to Event Signal/1 -> setAttribute/1
  Clock/1 -> Timed to Event Signal/1
  connections:
  OUT_Commodity/RConn1 -- setAttribute/RConn1
  Source/RConn1 -- setAttribute/LConn1

== system Distribution/Customer7/AggregateCommodity ==
  Clock : Clock
  Source : TimeBasedEntityGenerator  Distribution=Exponential  InitialSeed=49686  Mean=Mean  GenerateEntityAtSimulationStart=off
  Timed to Event Signal : TimedToEventSignal
  setAttribute : SetAttribute  AttributeName=Route|Origin|Destination|Start  AttributeFrom=Dialog|Dialog|Dialog|Signal port  AttributeValue=[1 0 1]|1|1|1  AttributeTreatAsVector=0|1|1|1  EvaluatedAttributeValue={ [1 0 1];1;1;[]}
      settings: InputPortMap=u3
  OUT_Commodity : PMIOPort  Side=Right
  wires:
  Timed to Event Signal/1 -> setAttribute/1
  Clock/1 -> Timed to Event Signal/1
  connections:
  OUT_Commodity/RConn1 -- setAttribute/RConn1
  Source/RConn1 -- setAttribute/LConn1

== system Distribution/Customer8/AggregateCommodity ==
  Clock : Clock
  Source : TimeBasedEntityGenerator  Distribution=Exponential  InitialSeed=52903  Mean=Mean  GenerateEntityAtSimulationStart=off
  Timed to Event Signal : TimedToEventSignal
  setAttribute : SetAttribute  AttributeName=Route|Origin|Destination|Start  AttributeFrom=Dialog|Dialog|Dialog|Signal port  AttributeValue=[1 0 1]|1|1|1  AttributeTreatAsVector=0|1|1|1  EvaluatedAttributeValue={ [1 0 1];1;1;[]}
      settings: InputPortMap=u3
  OUT_Commodity : PMIOPort  Side=Right
  wires:
  Timed to Event Signal/1 -> setAttribute/1
  Clock/1 -> Timed to Event Signal/1
  connections:
  OUT_Commodity/RConn1 -- setAttribute/RConn1
  Source/RConn1 -- setAttribute/LConn1

== system Distribution/Customer9/AggregateCommodity ==
  Clock : Clock
  Source : TimeBasedEntityGenerator  Distribution=Exponential  InitialSeed=56120  Mean=Mean  GenerateEntityAtSimulationStart=off
  Timed to Event Signal : TimedToEventSignal
  setAttribute : SetAttribute  AttributeName=Route|Origin|Destination|Start  AttributeFrom=Dialog|Dialog|Dialog|Signal port  AttributeValue=[1 0 1]|1|1|1  AttributeTreatAsVector=0|1|1|1  EvaluatedAttributeValue={ [1 0 1];1;1;[]}
      settings: InputPortMap=u3
  OUT_Commodity : PMIOPort  Side=Right
  wires:
  Timed to Event Signal/1 -> setAttribute/1
  Clock/1 -> Timed to Event Signal/1
  connections:
  OUT_Commodity/RConn1 -- setAttribute/RConn1
  Source/RConn1 -- setAttribute/LConn1

== system Distribution/Depot3/Resource_Pool ==
  Event-Based Entity Generator : EventBasedEntityGenerator  GenerateEntitiesUpon=Function call from port fcn
  FIFO Queue : FIFOQueue  Capacity=8
  Path Combiner : PathCombiner  NumberInputPorts=2
  Time-Based Function-Call Generator : TimeBasedFunctionCallGenerator  EventGenerationMode=Only at simulation start  NumberOfEventsPerPeriod=Quantity
  Acquire : PMIOPort  Side=Left
  Return : PMIOPort  Port=2  Side=Right
  wires:
  Time-Based Function-Call Generator/1 -> Event-Based Entity Generator/1
  connections:
  Acquire/RConn1 -- FIFO Queue/RConn1
  Return/RConn1 -- Path Combiner/LConn2
  Path Combiner/RConn1 -- FIFO Queue/LConn1
  Event-Based Entity Generator/RConn1 -- Path Combiner/LConn1
